simulink model "KUKA_LBR_Simulink_model_flatness_based_control"  (R2017a)
settings: Solver=VariableStepAuto  StartTime=0.0  StopTime=T  RelTol=1e-3
InitFcn:
  | main
values from neighbouring files (symbols this model uses):
  elbowAngle = elbowAngle * pi/180    (= 0)    [KUKA_LBR_init.m]    (also in Untitled2.m)
  KAnaJacNum = [k_ind 0 0 0 0 0 ;                 0  k_ind 0 0 0 0 ;                    0 0 k_ind 0 0 0 ;                      0 0 0 k_ind 0 0 ;                        0 0 0 0 k_ind 0 ;                          0 0 0 0 0 k_ind ;                            ]    [KUKA_LBR_init.m]
  Kuka_LBR_param_simu = Simulink.Parameter(Kuka_LBR_param_simu)    [KUKA_LBR_init.m]
  KUKA_LBR_x0 = [x1_0 x2_0 x3_0 x4_0 x5_0 x6_0 x7_0 x8_0 x9_0 x10_0 x11_0 x12_0 x13_0 x14_0]    [KUKA_LBR_init.m]
  rpyDes = rpyDes * pi/180    [KUKA_LBR_init.m]    (also in Untitled2.m)
  T = 0.5    [KUKA_LBR_init.m]
  vecGlobalConfig = [1; 1; 1]    [KUKA_LBR_init.m]    (also in Untitled2.m = [1, 1, 1])
undefined symbols (not defined in the file or in its folder): Kuka_LBR_param
(part 19 of 19)

== matlab function KUKA_LBR_Simulink_model_flatness_based_control/KUKA_LBR_forward_kinematic ==
  data: vecJointPos_ input; vecPosReal output; Kuka_LBR_param_ input
function vecPosReal = KUKA_LBR_forward_kinematic(vecJointPos_,Kuka_LBR_param_)

q1 = vecJointPos_(1);
q2 = vecJointPos_(2);
q3 = vecJointPos_(3);
q4 = vecJointPos_(4);
q5 = vecJointPos_(5);
q6 = vecJointPos_(6);
q7 = vecJointPos_(7);

T07 = [cos(q7).*(cos(q6).*(cos(q5).*(cos(q4).*(cos(q1).*cos(q2).*cos(q3)+(-1) ...
  .*sin(q1).*sin(q3))+cos(q1).*sin(q2).*sin(q4))+((-1).*cos(q3).*sin(q1)+( ...
  -1).*cos(q1).*cos(q2).*sin(q3)).*sin(q5))+((-1).*cos(q1).*cos(q4).*sin( ...
  q2)+(cos(q1).*cos(q2).*cos(q3)+(-1).*sin(q1).*sin(q3)).*sin(q4)).*sin( ...
  q6))+(cos(q5).*((-1).*cos(q3).*sin(q1)+(-1).*cos(q1).*cos(q2).*sin(q3))+ ...
  (-1).*(cos(q4).*(cos(q1).*cos(q2).*cos(q3)+(-1).*sin(q1).*sin(q3))+cos( ...
  q1).*sin(q2).*sin(q4)).*sin(q5)).*sin(q7),cos(q7).*(cos(q5).*((-1).*cos( ...
  q3).*sin(q1)+(-1).*cos(q1).*cos(q2).*sin(q3))+(-1).*(cos(q4).*(cos(q1).* ...
  cos(q2).*cos(q3)+(-1).*sin(q1).*sin(q3))+cos(q1).*sin(q2).*sin(q4)).* ...
  sin(q5))+(-1).*(cos(q6).*(cos(q5).*(cos(q4).*(cos(q1).*cos(q2).*cos(q3)+ ...
  (-1).*sin(q1).*sin(q3))+cos(q1).*sin(q2).*sin(q4))+((-1).*cos(q3).*sin( ...
  q1)+(-1).*cos(q1).*cos(q2).*sin(q3)).*sin(q5))+((-1).*cos(q1).*cos(q4).* ...
  sin(q2)+(cos(q1).*cos(q2).*cos(q3)+(-1).*sin(q1).*sin(q3)).*sin(q4)).* ...
  sin(q6)).*sin(q7),(-1).*cos(q6).*((-1).*cos(q1).*cos(q4).*sin(q2)+(cos( ...
  q1).*cos(q2).*cos(q3)+(-1).*sin(q1).*sin(q3)).*sin(q4))+(cos(q5).*(cos( ...
  q4).*(cos(q1).*cos(q2).*cos(q3)+(-1).*sin(q1).*sin(q3))+cos(q1).*sin(q2) ...
  .*sin(q4))+((-1).*cos(q3).*sin(q1)+(-1).*cos(q1).*cos(q2).*sin(q3)).* ...
  sin(q5)).*sin(q6),Kuka_LBR_param_.dblLink23Len.*cos(q1).*sin(q2)+Kuka_LBR_param_.dblLink45Len.*(cos(q1).*cos(q4).*sin(q2)+ ...
  (-1).*(cos(q1).*cos(q2).*cos(q3)+(-1).*sin(q1).*sin(q3)).*sin(q4))+Kuka_LBR_param_.dblLink67Len.* ...
  ((-1).*cos(q6).*((-1).*cos(q1).*cos(q4).*sin(q2)+(cos(q1).*cos(q2).*cos( ...
  q3)+(-1).*sin(q1).*sin(q3)).*sin(q4))+(cos(q5).*(cos(q4).*(cos(q1).*cos( ...
  q2).*cos(q3)+(-1).*sin(q1).*sin(q3))+cos(q1).*sin(q2).*sin(q4))+((-1).* ...
  cos(q3).*sin(q1)+(-1).*cos(q1).*cos(q2).*sin(q3)).*sin(q5)).*sin(q6)); ...
  cos(q7).*(cos(q6).*(cos(q5).*(cos(q4).*(cos(q2).*cos(q3).*sin(q1)+cos( ...
  q1).*sin(q3))+sin(q1).*sin(q2).*sin(q4))+(cos(q1).*cos(q3)+(-1).*cos(q2) ...
  .*sin(q1).*sin(q3)).*sin(q5))+((-1).*cos(q4).*sin(q1).*sin(q2)+(cos(q2) ...
  .*cos(q3).*sin(q1)+cos(q1).*sin(q3)).*sin(q4)).*sin(q6))+(cos(q5).*(cos( ...
  q1).*cos(q3)+(-1).*cos(q2).*sin(q1).*sin(q3))+(-1).*(cos(q4).*(cos(q2).* ...
  cos(q3).*sin(q1)+cos(q1).*sin(q3))+sin(q1).*sin(q2).*sin(q4)).*sin(q5)) ...
  .*sin(q7),cos(q7).*(cos(q5).*(cos(q1).*cos(q3)+(-1).*cos(q2).*sin(q1).* ...
  sin(q3))+(-1).*(cos(q4).*(cos(q2).*cos(q3).*sin(q1)+cos(q1).*sin(q3))+ ...
  sin(q1).*sin(q2).*sin(q4)).*sin(q5))+(-1).*(cos(q6).*(cos(q5).*(cos(q4) ...
  .*(cos(q2).*cos(q3).*sin(q1)+cos(q1).*sin(q3))+sin(q1).*sin(q2).*sin(q4) ...
  )+(cos(q1).*cos(q3)+(-1).*cos(q2).*sin(q1).*sin(q3)).*sin(q5))+((-1).* ...
  cos(q4).*sin(q1).*sin(q2)+(cos(q2).*cos(q3).*sin(q1)+cos(q1).*sin(q3)).* ...
  sin(q4)).*sin(q6)).*sin(q7),(-1).*cos(q6).*((-1).*cos(q4).*sin(q1).*sin( ...
  q2)+(cos(q2).*cos(q3).*sin(q1)+cos(q1).*sin(q3)).*sin(q4))+(cos(q5).*( ...
  cos(q4).*(cos(q2).*cos(q3).*sin(q1)+cos(q1).*sin(q3))+sin(q1).*sin(q2).* ...
  sin(q4))+(cos(q1).*cos(q3)+(-1).*cos(q2).*sin(q1).*sin(q3)).*sin(q5)).* ...
  sin(q6),Kuka_LBR_param_.dblLink23Len.*sin(q1).*sin(q2)+Kuka_LBR_param_.dblLink45Len.*(cos(q4).*sin(q1).*sin(q2)+(-1).*( ...
  cos(q2).*cos(q3).*sin(q1)+cos(q1).*sin(q3)).*sin(q4))+Kuka_LBR_param_.dblLink67Len.*((-1).*cos( ...
  q6).*((-1).*cos(q4).*sin(q1).*sin(q2)+(cos(q2).*cos(q3).*sin(q1)+cos(q1) ...
  .*sin(q3)).*sin(q4))+(cos(q5).*(cos(q4).*(cos(q2).*cos(q3).*sin(q1)+cos( ...
  q1).*sin(q3))+sin(q1).*sin(q2).*sin(q4))+(cos(q1).*cos(q3)+(-1).*cos(q2) ...
  .*sin(q1).*sin(q3)).*sin(q5)).*sin(q6));cos(q7).*(cos(q6).*(cos(q5).*(( ...
  -1).*cos(q3).*cos(q4).*sin(q2)+cos(q2).*sin(q4))+sin(q2).*sin(q3).*sin( ...
  q5))+((-1).*cos(q2).*cos(q4)+(-1).*cos(q3).*sin(q2).*sin(q4)).*sin(q6))+ ...
  (cos(q5).*sin(q2).*sin(q3)+(-1).*((-1).*cos(q3).*cos(q4).*sin(q2)+cos( ...
  q2).*sin(q4)).*sin(q5)).*sin(q7),cos(q7).*(cos(q5).*sin(q2).*sin(q3)+( ...
  -1).*((-1).*cos(q3).*cos(q4).*sin(q2)+cos(q2).*sin(q4)).*sin(q5))+(-1).* ...
  (cos(q6).*(cos(q5).*((-1).*cos(q3).*cos(q4).*sin(q2)+cos(q2).*sin(q4))+ ...
  sin(q2).*sin(q3).*sin(q5))+((-1).*cos(q2).*cos(q4)+(-1).*cos(q3).*sin( ...
  q2).*sin(q4)).*sin(q6)).*sin(q7),(-1).*cos(q6).*((-1).*cos(q2).*cos(q4)+ ...
  (-1).*cos(q3).*sin(q2).*sin(q4))+(cos(q5).*((-1).*cos(q3).*cos(q4).*sin( ...
  q2)+cos(q2).*sin(q4))+sin(q2).*sin(q3).*sin(q5)).*sin(q6),Kuka_LBR_param_.dblLink23Len.*cos(q2)+ ...
  Kuka_LBR_param_.dblLink45Len.*(cos(q2).*cos(q4)+cos(q3).*sin(q2).*sin(q4))+Kuka_LBR_param_.dblLink67Len.*((-1).*cos(q6).*( ...
  (-1).*cos(q2).*cos(q4)+(-1).*cos(q3).*sin(q2).*sin(q4))+(cos(q5).*((-1) ...
  .*cos(q3).*cos(q4).*sin(q2)+cos(q2).*sin(q4))+sin(q2).*sin(q3).*sin(q5)) ...
  .*sin(q6));0,0,0,1];

phibe = atan(T07(2,1)/T07(1,1));
thetabe = atan(T07(3,1)/sqrt(T07(3,2).^2+T07(3,3).^2));
psibe = atan(T07(3,2)/T07(3,3));

xdblTool = [Kuka_LBR_param_.dblToolLenX; Kuka_LBR_param_.dblToolLenY; Kuka_LBR_param_.dblToolLenZ; 1];
xbe      = T07*xdblTool;

vecPosReal = [xbe(1); xbe(2); xbe(3); phibe; thetabe; psibe]';

== matlab function KUKA_LBR_Simulink_model_flatness_based_control/KUKA_LBR_trajectotry_planning ==
  data: vecPosDes output; vecVelDes output; vecAccDes output; rpyDes_ input; quatOriDes output; t_ input; Kuka_LBR_param_ input; T_ input
function [vecPosDes, vecVelDes, vecAccDes, quatOriDes] = KUKA_LBR_trajectotry_planning(rpyDes_, t_, Kuka_LBR_param_,T_)
%Abbreviations for the various angular function

    xAngle = rpyDes_(1);
    yAngle = rpyDes_(2);
    zAngle = rpyDes_(3);


    cy = cos(zAngle * 0.5);
    sy = sin(zAngle * 0.5);
    cp = cos(yAngle * 0.5);
    sp = sin(yAngle * 0.5);
    cr = cos(xAngle * 0.5);
    sr = sin(xAngle * 0.5);

    q = [1 1 1 1];
    q(1) = cy * cp * cr + sy * sp * sr;
    q(2) = cy * cp * sr - sy * sp * cr;
    q(3) = sy * cp * sr + cy * sp * cr;
    q(4) = sy * cp * cr - cy * sp * sr;
    
    KUKA_length = Kuka_LBR_param_.dblLinkBase1Len + Kuka_LBR_param_.dblLink23Len + ...
                  Kuka_LBR_param_.dblLink45Len +  Kuka_LBR_param_.dblLink67Len; 
    
    x = KUKA_length/(3*sin(pi/6)*T_) * t_;
    y = 0;
    z = KUKA_length - (KUKA_length/3*T_) * t_;
    
    x_dot = (2*KUKA_length) / (3*T_);
    y_dot = 0;
    z_dot = - KUKA_length / (3*T_);
    
    x_ddot = 0;
    y_ddot = 0;
    z_ddot = 0;
    
vecPosDes  = [x y z];    
vecVelDes  = [x_dot y_dot z_dot];
vecAccDes  = [x_ddot y_ddot z_ddot];
quatOriDes = q;
